simulink model "oloop3"  (Simulink 10.0)
settings: Solver=ode45  StartTime=0.0  StopTime=120  MaxStep=1  RelTol=1e-3  AbsTol=1e-3
undefined symbols (not defined in the file): Aac, Bac, Cac, Dac
libraries: simulink3 x6, fdctools x3, fbuttons x2
settings Model: Creator=bhisma  LastModifiedBy=bhisma  ExtModeTrigMode=oneshot  ExtModeArmWhenConnect=off
settings DataIOCC: SignalLoggingSaveFormat=ModelDataLogs  SaveOutput=off  SaveTime=off  Refine=4
settings OptimizationCC: BlockReduction=off  BooleanDataType=off  LifeSpan=auto
settings DebuggingCC: SaveWithParameterizedLinksMsg=none  SignalResolutionControl=TryResolveAllWithWarning  MultiTaskDSMMsg=warning  MultiTaskCondExecSysMsg=none  SFUnexpectedBacktrackingDiag=error  SFNoUnconditionalDefaultTransitionDiag=error  SFExecutionAtInitializationDiag=warning  ArithmeticOperatorsInVariantConditions=error
settings HardwareCC: ProdBitPerPointer=64  ProdBitPerSizeT=64  ProdBitPerPtrDiffT=64  ProdLargestAtomicFloat=Float  ProdIntDivRoundTo=Zero  ProdEndianess=LittleEndian  ProdWordSize=64  ProdHWDeviceType=Intel->x86-64 (Windows64)  TargetUnknown=on
settings SFSimCC: SimUseLocalCustomCode=on  CustomCodeUndefinedFunction=FilterOut
settings RTWCC: TemplateMakefile=grt_vc.tmf  RTWUseLocalCustomCode=on
settings CodeAppCC: StateflowObjectComments=off
settings GRTTargetCC: TargetLangStandard=C99 (ISO)
settings ConfigComp: CovMetricSettings=dwe  CovHtmlReporting=off  CovSaveCumulativeToWorkspaceVar=off  CovSaveSingleToWorkspaceVar=off

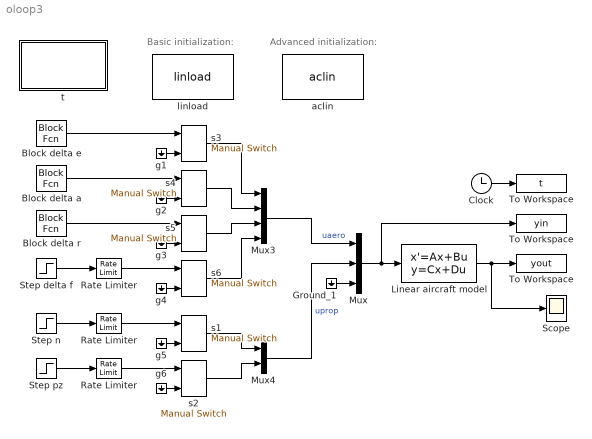
== system oloop3 ==
  note: Basic initialization:
  note: Advanced initialization:
  " Rate Limiter" : RateLimiter  RisingSlewLimit=1.0  FallingSlewLimit=-1.0
  " To Workspace  " : ToWorkspace  VariableName=yin
  Block delta a : fdctools/Block Fcn  yinit=0  yblock=3*pi/180  tstart=0.001  tstop=2
  Block delta e : fdctools/Block Fcn  yinit=0  yblock=3*pi/180  tstart=0.001  tstop=2
  Block delta r : fdctools/Block Fcn  yinit=0  yblock=3*pi/180  tstart=0.001  tstop=2
  Clock : Clock
  Ground_1 : Ground
  Linear aircraft model : StateSpace  A=Aac  B=Bac  C=Cac  D=Dac  InitialCondition=0
  Mux : Mux  Inputs=[4 2 6]
  Mux3 : Mux
  Mux4 : Mux  Inputs=2
  Rate Limiter : RateLimiter  RisingSlewLimit=pi/180  FallingSlewLimit=-pi/180
  "Rate Limiter " : RateLimiter  RisingSlewLimit=50  FallingSlewLimit=-50
  Scope : Scope
  Step delta f : Step  Time=0.001  After=3*pi/180  SampleTime=0
  Step n : Step  Time=0.001  After=200  SampleTime=0
  Step pz : Step  Time=0.001  After=2  SampleTime=0
  To Workspace : ToWorkspace  VariableName=t
  "To Workspace " : ToWorkspace  VariableName=yout
  aclin : fbuttons/aclin
  g{1..6} (6 alike) : Ground
  linload : fbuttons/linload
  s{1..2,4..6} (5 alike) : simulink3/Nonlinear/Manual Switch  sw=0  action=0
      settings: SourceProductName=Simulink  SourceProductBaseCode=SL
  s3 : simulink3/Nonlinear/Manual Switch  sw=1  action=0
      settings: SourceProductName=Simulink  SourceProductBaseCode=SL
  t : Subsystem
      settings: OpenFcn=browse oloop
      mask Display: disp('OLOOP3\nMarc Rauw\nJanuary 2004')
  wires:
  Step delta f/1 -> Rate Limiter/1
  g5/1 -> s1/2
  g6/1 -> s2/2
  g1/1 -> s3/2
  g4/1 -> s6/2
  g3/1 -> s5/2
  g2/1 -> s4/2
  s2/1 -> Mux4/2
  s1/1 -> Mux4/1
  s6/1 -> Mux3/4
  s5/1 -> Mux3/3
  s4/1 -> Mux3/2
  s3/1 -> Mux3/1
  Block delta e/1 -> s3/1
  Block delta a/1 -> s4/1
  Block delta r/1 -> s5/1
  Rate Limiter/1 -> s6/1
  Step n/1 -> "Rate Limiter "/1
  "Rate Limiter "/1 -> s1/1
  Step pz/1 -> " Rate Limiter"/1
  " Rate Limiter"/1 -> s2/1
  Clock/1 -> To Workspace/1
  Mux3/1 -> Mux/1  "uaero"
  Mux4/1 -> Mux/2  "uprop"
  Linear aircraft model/1 -> "To Workspace "/1, Scope/1
  Mux/1 -> Linear aircraft model/1, " To Workspace  "/1
  Ground_1/1 -> Mux/3

== system oloop3/t ==
